simulink model "TC1_MappingRing"  (R2016a)
settings: Solver=FixedStepAuto  StartTime=0.0  StopTime=10.0  RelTol=1e-3
model workspace: external: MAT-File TC1_MappingRing.mat (data not in the file)
values from neighbouring files (symbols this model uses):
  dripTestCasedripX = 0.19576554744588748    (= 0.195765547446)    [TC1_MappingSingle_params.m]
  dripTestCasedripY = 1.0533299169351737    (= 1.05332991694)    [TC1_MappingSingle_params.m]
libraries: libTLAsserts x6
settings Model: Creator=Josef  LastModifiedBy=Josef
settings GRTTargetCC: GeneratePreprocessorConditionals=Use local settings

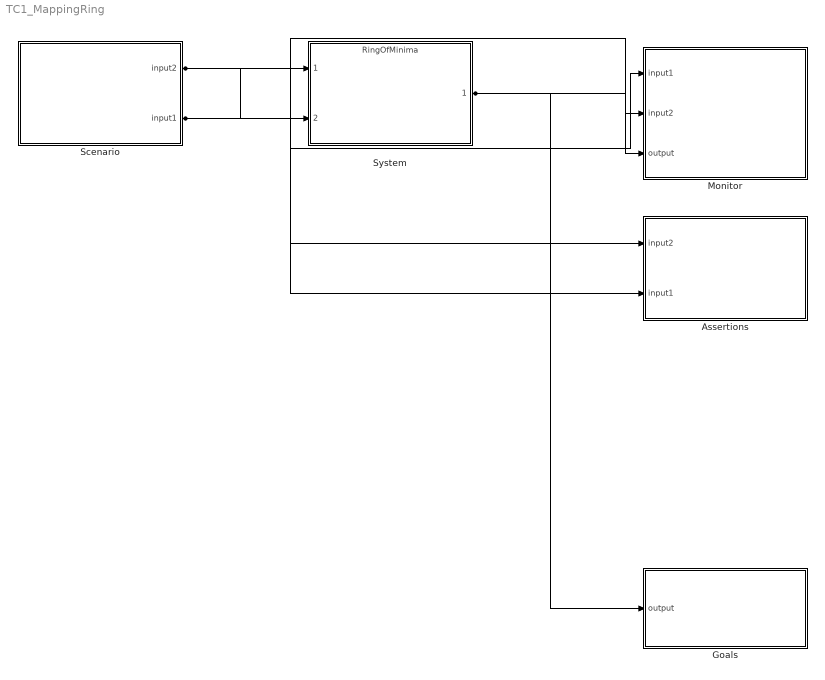
== system TC1_MappingRing ==
  Assertions : Subsystem
  Goals : Subsystem
  Monitor : Subsystem
  Scenario : Subsystem
  System : ModelReference  ModelNameDialog=RingOfMinima  SimulationMode=Normal  ModelReferenceVersion=1.7
  wires:
  Scenario/2(input1) -> System/1, Monitor/1(input1), Assertions/2(input1)
  Scenario/1(input2) -> System/2, Monitor/2(input2), Assertions/1(input2)
  System/1 -> Monitor/3(output), Goals/1(output)

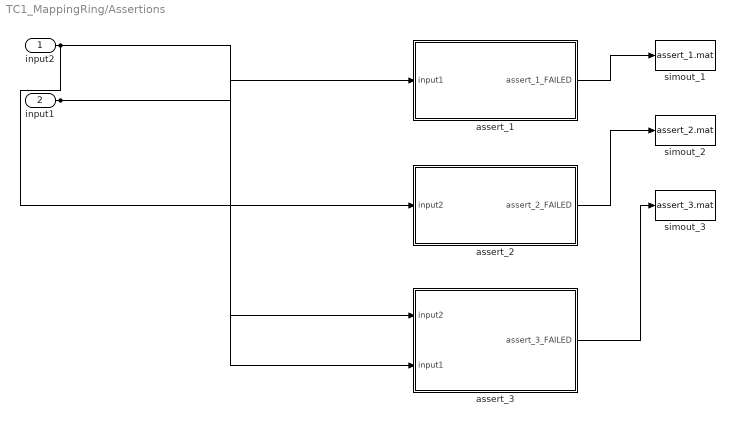
== system TC1_MappingRing/Assertions ==
  input2 : Inport
  input1 : Inport  Port=2
  assert_1 : Subsystem
  assert_2 : Subsystem
  assert_3 : Subsystem
  simout_1 : ToFile  Filename=assert_1.mat  MatrixName=assert_1  SaveFormat=Timeseries
  simout_2 : ToFile  Filename=assert_2.mat  MatrixName=assert_2  SaveFormat=Timeseries
  simout_3 : ToFile  Filename=assert_3.mat  MatrixName=assert_3  SaveFormat=Timeseries
  wires:
  input1/1 -> assert_1/1(input1), assert_3/2(input1)
  assert_1/1(assert_1_FAILED) -> simout_1/1
  input2/1 -> assert_2/1(input2), assert_3/1(input2)
  assert_2/1(assert_2_FAILED) -> simout_2/1
  assert_3/1(assert_3_FAILED) -> simout_3/1

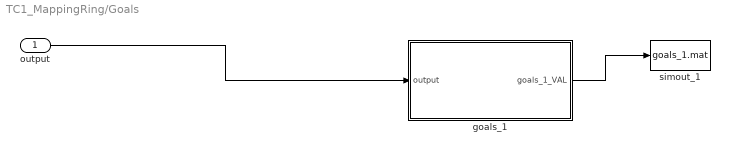
== system TC1_MappingRing/Goals ==
  output : Inport
  goals_1 : Subsystem
  simout_1 : ToFile  Filename=goals_1.mat  MatrixName=goals_1  SaveFormat=Timeseries
  wires:
  output/1 -> goals_1/1(output)
  goals_1/1(goals_1_VAL) -> simout_1/1

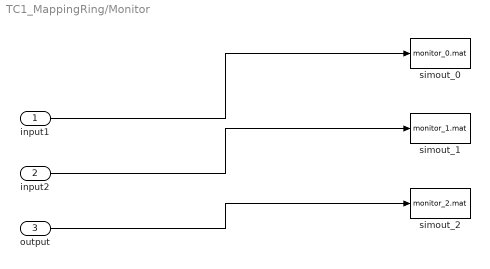
== system TC1_MappingRing/Monitor ==
  input1 : Inport
  input2 : Inport  Port=2
  output : Inport  Port=3
  simout_0 : ToFile  Filename=monitor_0.mat  MatrixName=input1  SaveFormat=Timeseries
  simout_1 : ToFile  Filename=monitor_1.mat  MatrixName=input2  SaveFormat=Timeseries
  simout_2 : ToFile  Filename=monitor_2.mat  MatrixName=output  SaveFormat=Timeseries
  wires:
  input1/1 -> simout_0/1
  input2/1 -> simout_1/1
  output/1 -> simout_2/1

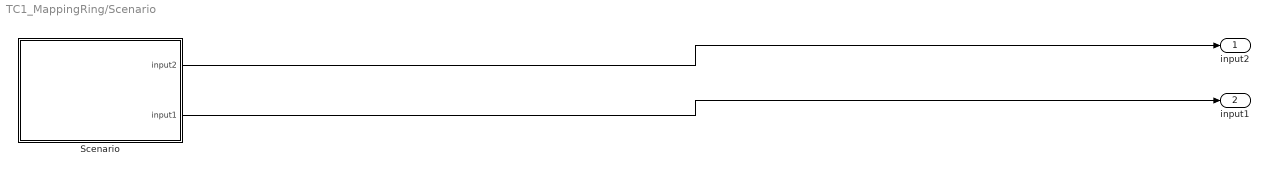
== system TC1_MappingRing/Scenario ==
  Scenario : Stateflow chart  TreatAsAtomicUnit=on
  input2 : Outport
  input1 : Outport  Port=2
  wires:
  Scenario/2(input1) -> input1/1
  Scenario/1(input2) -> input2/1

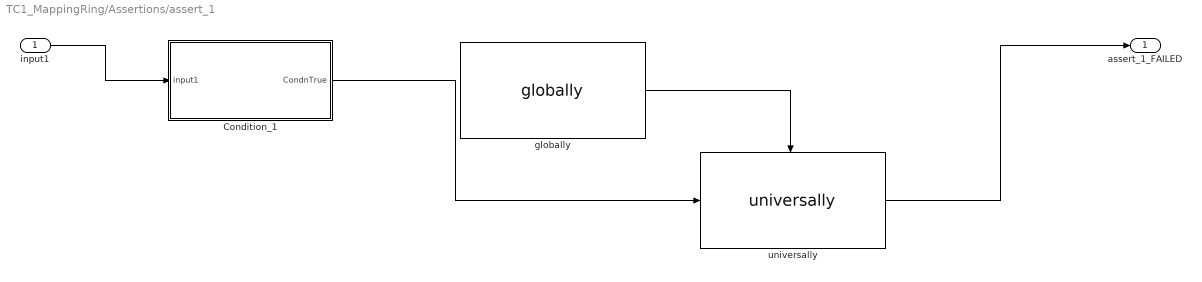
== system TC1_MappingRing/Assertions/assert_1 ==
  input1 : Inport
  Condition_1 : Subsystem
  globally : libTLAsserts/globally
  universally : libTLAsserts/universally
  assert_1_FAILED : Outport
  wires:
  input1/1 -> Condition_1/1(input1)
  Condition_1/1(CondnTrue) -> universally/1
  globally/1 -> universally/Enable
  universally/1 -> assert_1_FAILED/1

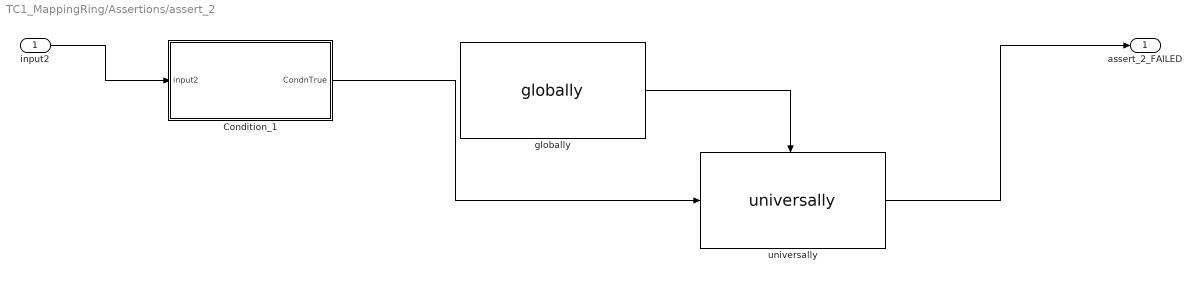
== system TC1_MappingRing/Assertions/assert_2 ==
  input2 : Inport
  Condition_1 : Subsystem
  globally : libTLAsserts/globally
  universally : libTLAsserts/universally
  assert_2_FAILED : Outport
  wires:
  input2/1 -> Condition_1/1(input2)
  Condition_1/1(CondnTrue) -> universally/1
  globally/1 -> universally/Enable
  universally/1 -> assert_2_FAILED/1

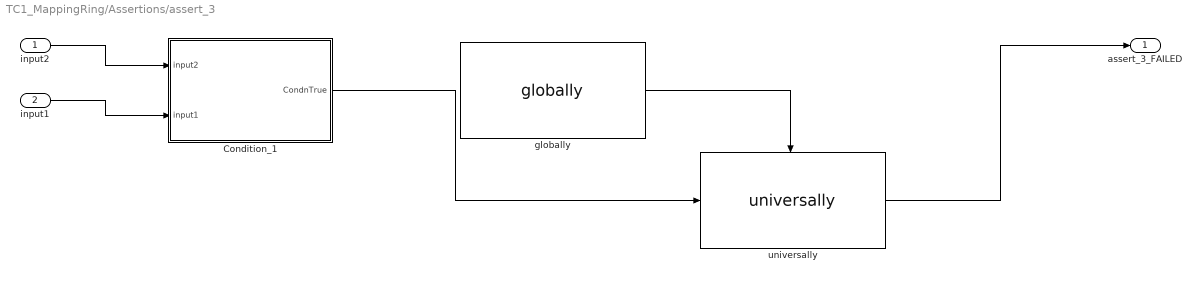
== system TC1_MappingRing/Assertions/assert_3 ==
  input2 : Inport
  input1 : Inport  Port=2
  Condition_1 : Subsystem
  globally : libTLAsserts/globally
  universally : libTLAsserts/universally
  assert_3_FAILED : Outport
  wires:
  input2/1 -> Condition_1/1(input2)
  input1/1 -> Condition_1/2(input1)
  Condition_1/1(CondnTrue) -> universally/1
  globally/1 -> universally/Enable
  universally/1 -> assert_3_FAILED/1

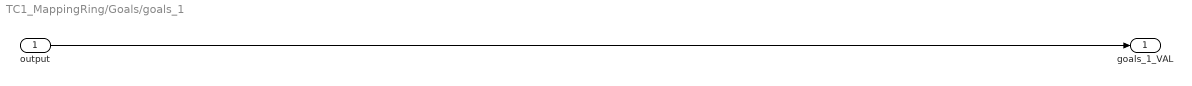
== system TC1_MappingRing/Goals/goals_1 ==
  output : Inport
  goals_1_VAL : Outport
  wires:
  output/1 -> goals_1_VAL/1

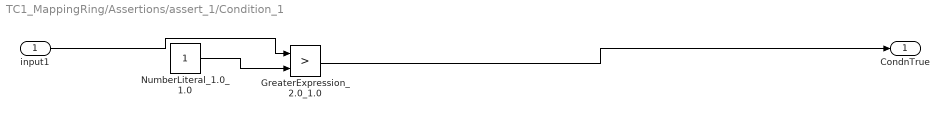
== system TC1_MappingRing/Assertions/assert_1/Condition_1 ==
  input1 : Inport
  GreaterExpression_2.0_1.0 : RelationalOperator  Operator=>  OutDataTypeStr=boolean
  NumberLiteral_1.0_1.0 : Constant
  CondnTrue : Outport
  wires:
  input1/1 -> GreaterExpression_2.0_1.0/1
  NumberLiteral_1.0_1.0/1 -> GreaterExpression_2.0_1.0/2
  GreaterExpression_2.0_1.0/1 -> CondnTrue/1

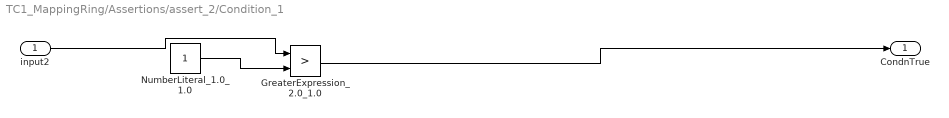
== system TC1_MappingRing/Assertions/assert_2/Condition_1 ==
  input2 : Inport
  GreaterExpression_2.0_1.0 : RelationalOperator  Operator=>  OutDataTypeStr=boolean
  NumberLiteral_1.0_1.0 : Constant
  CondnTrue : Outport
  wires:
  input2/1 -> GreaterExpression_2.0_1.0/1
  NumberLiteral_1.0_1.0/1 -> GreaterExpression_2.0_1.0/2
  GreaterExpression_2.0_1.0/1 -> CondnTrue/1

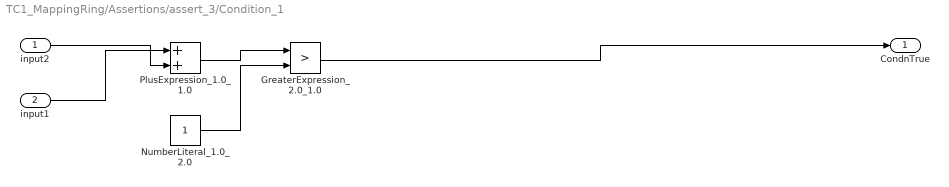
== system TC1_MappingRing/Assertions/assert_3/Condition_1 ==
  input2 : Inport
  input1 : Inport  Port=2
  GreaterExpression_2.0_1.0 : RelationalOperator  Operator=>  OutDataTypeStr=boolean
  NumberLiteral_1.0_2.0 : Constant
  PlusExpression_1.0_1.0 : Sum
  CondnTrue : Outport
  wires:
  input1/1 -> PlusExpression_1.0_1.0/1
  input2/1 -> PlusExpression_1.0_1.0/2
  PlusExpression_1.0_1.0/1 -> GreaterExpression_2.0_1.0/1
  NumberLiteral_1.0_2.0/1 -> GreaterExpression_2.0_1.0/2
  GreaterExpression_2.0_1.0/1 -> CondnTrue/1

== stateflow chart TC1_MappingRing/Scenario/Scenario ==
  state Act_A_Step1
    entry: input1 = dripTestCasedripX;
    entry: input2 = dripTestCasedripY;
  (default) -> Act_A_Step1
  data: input2 output; input1 output; dripTestCasedripY parameter; dripTestCasedripX parameter
